simulink model "ejercicio_6d"  (R2020a)
settings: Solver=ode45  StartTime=0.0  StopTime=1  MaxStep=1e-4  RelTol=1e-5
model workspace: external: MATLAB File D:\Ferran\Facultad\UNCuyo\Meca\Automática y Máquinas Eléctricas\Proyecto final\matlab\parametros_y_especs\parametros_y_especif.m (data not in the file)
undefined symbols (not defined in the file): alpha_Cu, beq, Cts, Jeq, L_ls, lambda_m, Ld, Lq, Pp, r, Rref, Rts_amb, sigbuilder_block, Tref
settings Model: Creator=Ferran  LastModifiedBy=Ferran

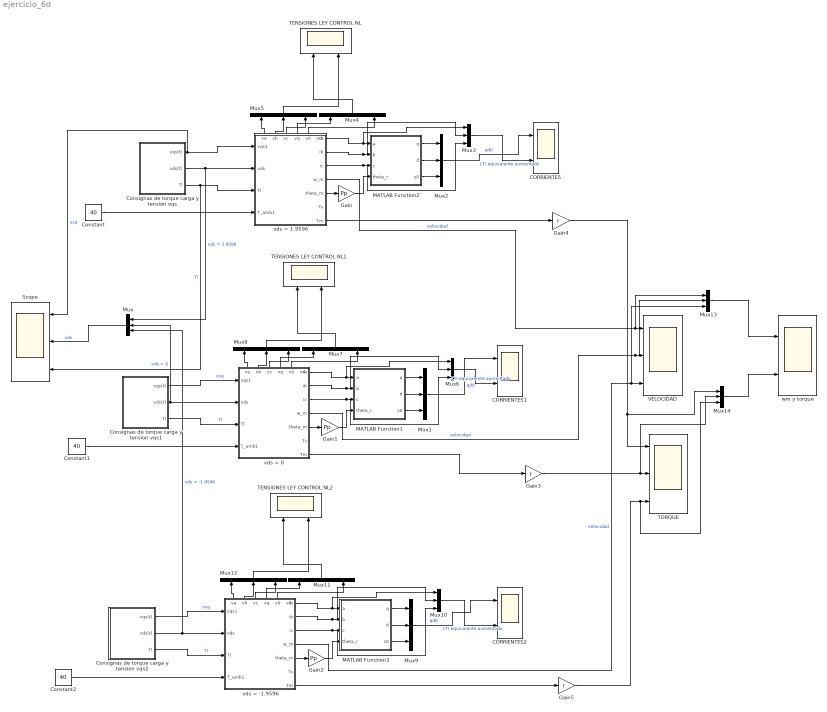
== system ejercicio_6d ==
  CORRIENTES : Scope  NumInputPorts=2
  CORRIENTES1 : Scope  NumInputPorts=2
  CORRIENTES2 : Scope  NumInputPorts=2
  Consignas de torque carga y tension vqs : Subsystem  Tag=STV Subsys  LoadFcn=sigbuilder_block('load');  StartFcn=sigbuilder_block('start');  StopFcn=sigbuilder_block('stop');  ClipboardFcn=sigbuilder_block('clipboard');  mask(Sigbuilder block){tuvar=[0:10]}
      mask help: Simulink:masks:SigbuilderBlock_MD
      mask init:
      | if ~strcmp(get_param(bdroot(gcbh),'SimulationStatus'),'stopped') tuvar = sigbuilder_block('maskInit'); end
      settings: CopyFcn=sigbuilder_block('copy');  DeleteFcn=sigbuilder_block('delete');  ModelCloseFcn=sigbuilder_block('modelClose');  PreSaveFcn=sigbuilder_block('preSave');  PauseFcn=sigbuilder_block('pause');  ContinueFcn=sigbuilder_block('continue');  NameChangeFcn=sigbuilder_block('namechange');  OpenFcn=sigbuilder_block('open',[352.2 100.2 550.8 400.2 ]);  CloseFcn=sigbuilder_block('close');
      mask Display: plot(0, 0, 100, 100,[2, 2, 32, 32, 2], [68, 8, 8, 68, 68],[32, 2], [38, 38], [32, 19, 2],[53, 60, 44], [32, 17, 17, 2],[16, 16, 31, 31]);txt = getActiveGroup(gcbh);text(2, 100, txt,'verticalAlignment', 'top');
  Consignas de torque carga y tension vqs1 : Subsystem  Tag=STV Subsys  LoadFcn=sigbuilder_block('load');  StartFcn=sigbuilder_block('start');  StopFcn=sigbuilder_block('stop');  ClipboardFcn=sigbuilder_block('clipboard');  mask(Sigbuilder block){tuvar=[0:10]}
      mask help: Simulink:masks:SigbuilderBlock_MD
      mask init:
      | if ~strcmp(get_param(bdroot(gcbh),'SimulationStatus'),'stopped') tuvar = sigbuilder_block('maskInit'); end
      settings: CopyFcn=sigbuilder_block('copy');  DeleteFcn=sigbuilder_block('delete');  ModelCloseFcn=sigbuilder_block('modelClose');  PreSaveFcn=sigbuilder_block('preSave');  PauseFcn=sigbuilder_block('pause');  ContinueFcn=sigbuilder_block('continue');  NameChangeFcn=sigbuilder_block('namechange');  OpenFcn=sigbuilder_block('open',[352.2 100.2 550.8 400.2 ]);  CloseFcn=sigbuilder_block('close');
      mask Display: plot(0, 0, 100, 100,[2, 2, 32, 32, 2], [68, 8, 8, 68, 68],[32, 2], [38, 38], [32, 19, 2],[53, 60, 44], [32, 17, 17, 2],[16, 16, 31, 31]);txt = getActiveGroup(gcbh);text(2, 100, txt,'verticalAlignment', 'top');
  Consignas de torque carga y tension vqs2 : Subsystem  Tag=STV Subsys  LoadFcn=sigbuilder_block('load');  StartFcn=sigbuilder_block('start');  StopFcn=sigbuilder_block('stop');  ClipboardFcn=sigbuilder_block('clipboard');  mask(Sigbuilder block){tuvar=[0:10]}
      mask help: Simulink:masks:SigbuilderBlock_MD
      mask init:
      | if ~strcmp(get_param(bdroot(gcbh),'SimulationStatus'),'stopped') tuvar = sigbuilder_block('maskInit'); end
      settings: CopyFcn=sigbuilder_block('copy');  DeleteFcn=sigbuilder_block('delete');  ModelCloseFcn=sigbuilder_block('modelClose');  PreSaveFcn=sigbuilder_block('preSave');  PauseFcn=sigbuilder_block('pause');  ContinueFcn=sigbuilder_block('continue');  NameChangeFcn=sigbuilder_block('namechange');  OpenFcn=sigbuilder_block('open',[352.2 100.2 550.8 400.2 ]);  CloseFcn=sigbuilder_block('close');
      mask Display: plot(0, 0, 100, 100,[2, 2, 32, 32, 2], [68, 8, 8, 68, 68],[32, 2], [38, 38], [32, 19, 2],[53, 60, 44], [32, 17, 17, 2],[16, 16, 31, 31]);txt = getActiveGroup(gcbh);text(2, 100, txt,'verticalAlignment', 'top');
  Constant : Constant  Value=40
  Constant1 : Constant  Value=40
  Constant2 : Constant  Value=40
  Gain : Gain  Gain=Pp
  Gain1 : Gain  Gain=Pp
  Gain2 : Gain  Gain=Pp
  Gain3 : Gain  Gain=r
  Gain4 : Gain  Gain=r
  Gain5 : Gain  Gain=r
  MATLAB Function1 : MATLAB Function  TreatAsAtomicUnit=on
  MATLAB Function2 : MATLAB Function  TreatAsAtomicUnit=on
  MATLAB Function3 : MATLAB Function  TreatAsAtomicUnit=on
  Mux{,1..14} (15 alike) : Mux  Inputs=3
  Scope : Scope  NumInputPorts=3
  TENSIONES LEY CONTROL NL : Scope  NumInputPorts=2
  TENSIONES LEY CONTROL NL1 : Scope  NumInputPorts=2
  TENSIONES LEY CONTROL NL2 : Scope  NumInputPorts=2
  TORQUE : Scope  NumInputPorts=3
  VELOCIDAD : Scope  NumInputPorts=3
  vds = -1.9596 : Subsystem
      settings: PortSchema="{\"entries\":[{\"content\":{\"sides\":[{\"content\":{\"connectorIds\":[\"In1\",\"In2\",\"In3\",\"In4\"]},\"type\":\"ConnectorPlacement.EquallySpacedRectSide\",\"uuid\":\"b8095cac-d600-4a62-9325-3b74ef7eef83\"},{\"content\":{\"connectorIds\":[\"Out1\",\"Out2\",\"Out3\",\"Out4\",\"Out5\",\"Out6\",\"Out7\"],\"side\":\"RIGHT\"},\"type\":\"ConnectorPlacement.EquallySpacedRectSide\",\"uuid\":\"fc0a756d-ae96-4315-bbed-bdc2bfc1e608\"},{\"content\":{\"connectorIds\":[\"Out8\",\"Out9\",\"Out10\",\"Out11\",\"Out12\",\"Out13\"],\"side\":\"TOP\"},\"type\":\"ConnectorPlacement.EquallySpacedRectSide\",\"uuid\":\"afbbfdf4-b2ca-493d-b8c6-50a451d76509\"}]},\"type\":\"ConnectorPlacement.EquallySpacedConnector\",\"uuid\":\"0b98ede1-47d2-4348-94af-35dda2463f57\"}],\"packageUris\":[\"http://schema.mathworks.com/mf0/Connector/19700101\"],\"version\":\"1.0\"}"
  vds = 0 : Subsystem
      settings: PortSchema="{\"entries\":[{\"content\":{\"sides\":[{\"content\":{\"connectorIds\":[\"In1\",\"In2\",\"In3\",\"In4\"]},\"type\":\"ConnectorPlacement.EquallySpacedRectSide\",\"uuid\":\"b8095cac-d600-4a62-9325-3b74ef7eef83\"},{\"content\":{\"connectorIds\":[\"Out1\",\"Out2\",\"Out3\",\"Out4\",\"Out5\",\"Out6\",\"Out7\"],\"side\":\"RIGHT\"},\"type\":\"ConnectorPlacement.EquallySpacedRectSide\",\"uuid\":\"fc0a756d-ae96-4315-bbed-bdc2bfc1e608\"},{\"content\":{\"connectorIds\":[\"Out8\",\"Out9\",\"Out10\",\"Out11\",\"Out12\",\"Out13\"],\"side\":\"TOP\"},\"type\":\"ConnectorPlacement.EquallySpacedRectSide\",\"uuid\":\"afbbfdf4-b2ca-493d-b8c6-50a451d76509\"}]},\"type\":\"ConnectorPlacement.EquallySpacedConnector\",\"uuid\":\"0b98ede1-47d2-4348-94af-35dda2463f57\"}],\"packageUris\":[\"http://schema.mathworks.com/mf0/Connector/19700101\"],\"version\":\"1.0\"}"
  vds = 1.9596 : Subsystem
      settings: PortSchema="{\"entries\":[{\"content\":{\"sides\":[{\"content\":{\"connectorIds\":[\"In1\",\"In2\",\"In3\",\"In4\"]},\"type\":\"ConnectorPlacement.EquallySpacedRectSide\",\"uuid\":\"b8095cac-d600-4a62-9325-3b74ef7eef83\"},{\"content\":{\"connectorIds\":[\"Out1\",\"Out2\",\"Out3\",\"Out4\",\"Out5\",\"Out6\",\"Out7\"],\"side\":\"RIGHT\"},\"type\":\"ConnectorPlacement.EquallySpacedRectSide\",\"uuid\":\"fc0a756d-ae96-4315-bbed-bdc2bfc1e608\"},{\"content\":{\"connectorIds\":[\"Out8\",\"Out9\",\"Out10\",\"Out11\",\"Out12\",\"Out13\"],\"side\":\"TOP\"},\"type\":\"ConnectorPlacement.EquallySpacedRectSide\",\"uuid\":\"afbbfdf4-b2ca-493d-b8c6-50a451d76509\"}]},\"type\":\"ConnectorPlacement.EquallySpacedConnector\",\"uuid\":\"0b98ede1-47d2-4348-94af-35dda2463f57\"}],\"packageUris\":[\"http://schema.mathworks.com/mf0/Connector/19700101\"],\"version\":\"1.0\"}"
  wm y torque : Scope  NumInputPorts=2
  wires:
  Constant/1 -> vds = 1.9596/4(T_amb1)
  Consignas de torque carga y tension vqs/1(vqs(t)) -> Scope/1, vds = 1.9596/1(vqs1)  "vsq"
  Consignas de torque carga y tension vqs/3(Tl) -> Scope/3, vds = 1.9596/3(Tl)  "Tl"
  MATLAB Function2/1(q) -> Mux2/1
  MATLAB Function2/2(d) -> Mux2/2
  MATLAB Function2/3(z0) -> Mux2/3
  vds = 1.9596/11(vq) -> Mux4/1
  vds = 1.9596/12(v0) -> Mux4/3
  Mux4/1 -> TENSIONES LEY CONTROL NL/1
  vds = 1.9596/8(va) -> Mux5/1
  vds = 1.9596/9(vb) -> Mux5/2
  vds = 1.9596/10(vc) -> Mux5/3
  Mux5/1 -> TENSIONES LEY CONTROL NL/2
  Consignas de torque carga y tension vqs/2(vds(t)) -> Mux/1, vds = 1.9596/2(vds)  "vds = 1.9596"
  vds = 1.9596/5(theta_m) -> Gain/1
  Gain/1 -> MATLAB Function2/4(theta_r)
  vds = 1.9596/1(ia) -> Mux3/1, MATLAB Function2/1(a)
  vds = 1.9596/2(ib) -> Mux3/2, MATLAB Function2/2(b)
  vds = 1.9596/3(ic) -> Mux3/3, MATLAB Function2/3(c)
  vds = 0/1(ia) -> Mux6/1, MATLAB Function1/1(a)
  MATLAB Function1/1(q) -> Mux1/1
  vds = 0/3(ic) -> Mux6/3, MATLAB Function1/3(c)
  vds = 0/5(theta_m) -> Gain1/1
  vds = 0/12(v0) -> Mux7/3
  Gain1/1 -> MATLAB Function1/4(theta_r)
  Consignas de torque carga y tension vqs1/2(vds(t)) -> Mux/2, vds = 0/2(vds)  "vds = 0"
  vds = 0/10(vc) -> Mux8/3
  Mux8/1 -> TENSIONES LEY CONTROL NL1/2
  vds = 0/2(ib) -> Mux6/2, MATLAB Function1/2(b)
  vds = 0/9(vb) -> Mux8/2
  Mux7/1 -> TENSIONES LEY CONTROL NL1/1
  vds = 0/11(vq) -> Mux7/1
  vds = 0/8(va) -> Mux8/1
  MATLAB Function1/3(z0) -> Mux1/3
  MATLAB Function1/2(d) -> Mux1/2
  Constant1/1 -> vds = 0/4(T_amb1)
  Consignas de torque carga y tension vqs1/3(Tl) -> vds = 0/3(Tl)  "Tl"
  Consignas de torque carga y tension vqs1/1(vqs(t)) -> vds = 0/1(vqs1)  "vsq"
  vds = -1.9596/1(ia) -> Mux10/1, MATLAB Function3/1(a)
  MATLAB Function3/1(q) -> Mux9/1
  vds = -1.9596/3(ic) -> Mux10/3, MATLAB Function3/3(c)
  vds = -1.9596/5(theta_m) -> Gain2/1
  vds = -1.9596/12(v0) -> Mux11/3
  Gain2/1 -> MATLAB Function3/4(theta_r)
  Consignas de torque carga y tension vqs2/2(vds(t)) -> Mux/3, vds = -1.9596/2(vds)  "vds = -1.9596"
  vds = -1.9596/10(vc) -> Mux12/3
  Mux12/1 -> TENSIONES LEY CONTROL NL2/2
  vds = -1.9596/2(ib) -> Mux10/2, MATLAB Function3/2(b)
  vds = -1.9596/9(vb) -> Mux12/2
  Mux11/1 -> TENSIONES LEY CONTROL NL2/1
  vds = -1.9596/11(vq) -> Mux11/1
  vds = -1.9596/8(va) -> Mux12/1
  MATLAB Function3/3(z0) -> Mux9/3
  MATLAB Function3/2(d) -> Mux9/2
  Constant2/1 -> vds = -1.9596/4(T_amb1)
  Consignas de torque carga y tension vqs2/3(Tl) -> vds = -1.9596/3(Tl)  "Tl"
  Consignas de torque carga y tension vqs2/1(vqs(t)) -> vds = -1.9596/1(vqs1)  "vsq"
  Mux/1 -> Scope/2  "vds"
  vds = 0/4(w_m) -> Mux13/2, VELOCIDAD/2  "velocidad"
  vds = 1.9596/4(w_m) -> Mux13/1, VELOCIDAD/1  "velocidad"
  vds = -1.9596/4(w_m) -> VELOCIDAD/3, Mux13/3  "velocidad"
  vds = 1.9596/7(Tm) -> Gain4/1
  vds = 0/7(Tm) -> Gain3/1
  vds = -1.9596/7(Tm) -> Gain5/1
  Mux13/1 -> wm y torque/1
  Mux14/1 -> wm y torque/2
  Mux3/1 -> CORRIENTES/2  "LTI equivalente aumentado"
  Mux2/1 -> CORRIENTES/1  "qd0"
  Mux6/1 -> CORRIENTES1/2  "LTI equivalente aumentado"
  Mux1/1 -> CORRIENTES1/1  "qd0"
  Mux10/1 -> CORRIENTES2/2  "LTI equivalente aumentado"
  Mux9/1 -> CORRIENTES2/1  "qd0"
  Gain3/1 -> Mux14/2, TORQUE/2
  Gain4/1 -> Mux14/1, TORQUE/1
  Gain5/1 -> Mux14/3, TORQUE/3

== system ejercicio_6d/Consignas de torque carga y tension vqs ==
  Demux : Demux  Tag=STV Demux  Outputs=3
      settings: DisplayOption=none
  FromWs : FromWorkspace  Tag=STV FromWs  VariableName=tuvar
      SigBuilderData=|
      | common.afterFinalStr = 'Extrapolate'
      | common.sampleTime = 0
      | dataSet.timeRange = [0 2]
      | dataSet.name = 'Group 1'
      | sbobj.Groups.Name = 'Group 1'
      | sbobj.Groups.Signals(1).Name = 'vqs(t)'
      | sbobj.Groups.Signals(1).XData = [0 0.1 0.1 0.7 0.7 2]
      | sbobj.Groups.Signals(1).YData = [0 0 19.596 19.596 0 0]
      | sbobj.Groups.Signals(2).Name = 'vds(t)'
      | sbobj.Groups.Signals(2).XData = [0 0.5 0.5 2]
      | sbobj.Groups.Signals(2).YData = [0 0 1.9596 1.9596]
      | sbobj.Groups.Signals(3).Name = 'Tl'
      | sbobj.Groups.Signals(3).XData = [0 0.3 0.3 0.5 0.5 0.9 0.9 2]
      | sbobj.Groups.Signals(3).YData = [0 0 6.28 6.28 -6.28 -6.28 0 0]
      | sbobj.Groups.TimeRange = [0 2]
  vqs(t) : Outport  Tag=STV Outport
  vds(t) : Outport  Tag=STV Outport  Port=2
  Tl : Outport  Tag=STV Outport  Port=3
  wires:
  FromWs/1 -> Demux/1
  Demux/1 -> vqs(t)/1
  Demux/2 -> vds(t)/1
  Demux/3 -> Tl/1

== system ejercicio_6d/Consignas de torque carga y tension vqs1 ==
  Demux : Demux  Tag=STV Demux  Outputs=3
      settings: DisplayOption=none
  FromWs : FromWorkspace  Tag=STV FromWs  VariableName=tuvar
      SigBuilderData=|
      | common.afterFinalStr = 'Extrapolate'
      | common.sampleTime = 0
      | dataSet.timeRange = [0 2]
      | dataSet.name = 'Group 1'
      | sbobj.Groups.Name = 'Group 1'
      | sbobj.Groups.Signals(1).Name = 'vqs(t)'
      | sbobj.Groups.Signals(1).XData = [0 0.1 0.1 0.7 0.7 2]
      | sbobj.Groups.Signals(1).YData = [0 0 19.596 19.596 0 0]
      | sbobj.Groups.Signals(2).Name = 'vds(t)'
      | sbobj.Groups.Signals(2).XData = [0 2]
      | sbobj.Groups.Signals(2).YData = [0 0]
      | sbobj.Groups.Signals(3).Name = 'Tl'
      | sbobj.Groups.Signals(3).XData = [0 0.3 0.3 0.5 0.5 0.9 0.9 2]
      | sbobj.Groups.Signals(3).YData = [0 0 6.28 6.28 -6.28 -6.28 0 0]
      | sbobj.Groups.TimeRange = [0 2]
  vqs(t) : Outport  Tag=STV Outport
  vds(t) : Outport  Tag=STV Outport  Port=2
  Tl : Outport  Tag=STV Outport  Port=3
  wires:
  FromWs/1 -> Demux/1
  Demux/1 -> vqs(t)/1
  Demux/2 -> vds(t)/1
  Demux/3 -> Tl/1

== system ejercicio_6d/Consignas de torque carga y tension vqs2 ==
  Demux : Demux  Tag=STV Demux  Outputs=3
      settings: DisplayOption=none
  FromWs : FromWorkspace  Tag=STV FromWs  VariableName=tuvar
      SigBuilderData=|
      | common.afterFinalStr = 'Extrapolate'
      | common.sampleTime = 0
      | dataSet.timeRange = [0 2]
      | dataSet.name = 'Group 1'
      | sbobj.Groups.Name = 'Group 1'
      | sbobj.Groups.Signals(1).Name = 'vqs(t)'
      | sbobj.Groups.Signals(1).XData = [0 0.1 0.1 0.7 0.7 2]
      | sbobj.Groups.Signals(1).YData = [0 0 19.596 19.596 0 0]
      | sbobj.Groups.Signals(2).Name = 'vds(t)'
      | sbobj.Groups.Signals(2).XData = [0 0.5 0.5 2]
      | sbobj.Groups.Signals(2).YData = [0 0 -1.9596 -1.9596]
      | sbobj.Groups.Signals(3).Name = 'Tl'
      | sbobj.Groups.Signals(3).XData = [0 0.3 0.3 0.5 0.5 0.9 0.9 2]
      | sbobj.Groups.Signals(3).YData = [0 0 6.28 6.28 -6.28 -6.28 0 0]
      | sbobj.Groups.TimeRange = [0 2]
  vqs(t) : Outport  Tag=STV Outport
  vds(t) : Outport  Tag=STV Outport  Port=2
  Tl : Outport  Tag=STV Outport  Port=3
  wires:
  FromWs/1 -> Demux/1
  Demux/1 -> vqs(t)/1
  Demux/2 -> vds(t)/1
  Demux/3 -> Tl/1

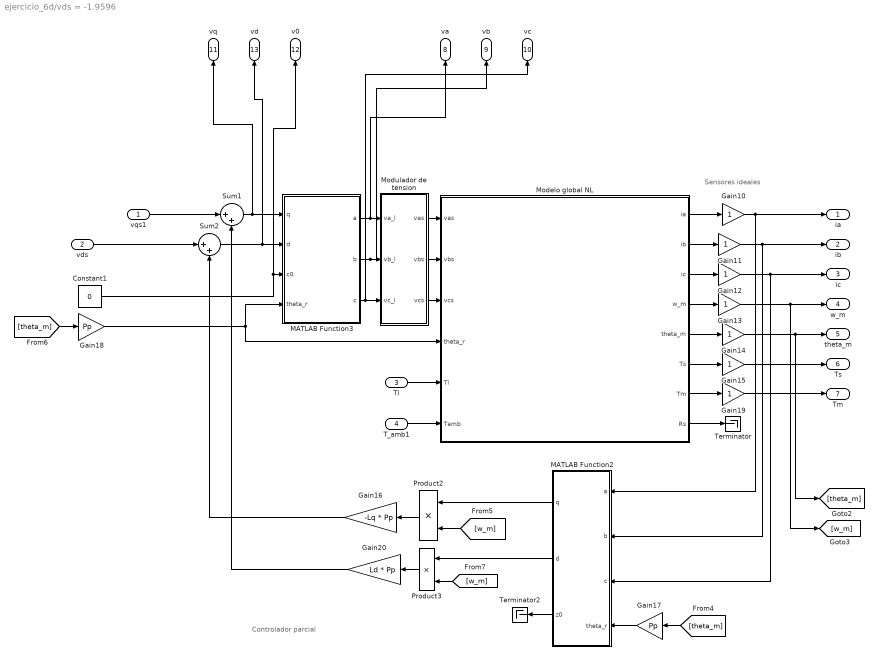
== system ejercicio_6d/vds = -1.9596 ==
  note: Sensores ideales
  note: Controlador parcial
  vqs1 : Inport
  vds : Inport  Port=2
  Tl : Inport  Port=3
  T_amb1 : Inport  Port=4
  Constant1 : Constant  Value=0
  Gain{10..15,19} (7 alike) : Gain
  Gain16 : Gain  Gain=-Lq * Pp
  Gain17 : Gain  Gain=Pp
  Gain18 : Gain  Gain=Pp
  Gain20 : Gain  Gain=Ld * Pp
  MATLAB Function2 : MATLAB Function  TreatAsAtomicUnit=on
  MATLAB Function3 : MATLAB Function  TreatAsAtomicUnit=on
  Modelo global NL : Subsystem
  Modulador de tension : Subsystem
  Product2 : Product
  Product3 : Product
  Sum1 : Sum  Inputs=|++
  Sum2 : Sum  Inputs=|++
  Terminator : Terminator
  Terminator2 : Terminator
  ia : Outport
  ib : Outport  Port=2
  ic : Outport  Port=3
  w_m : Outport  Port=4
  theta_m : Outport  Port=5
  Ts : Outport  Port=6
  Tm : Outport  Port=7
  va : Outport  Port=8
  vb : Outport  Port=9
  vc : Outport  Port=10
  vq : Outport  Port=11
  v0 : Outport  Port=12
  vd : Outport  Port=13
  wires:
  Modelo global NL/2(ib) -> Gain11/1
  MATLAB Function2/3(z0) -> Terminator2/1
  Modelo global NL/8(Rs) -> Terminator/1
  MATLAB Function2/2(d) -> Product3/1
  Modulador de tension/3(vcs) -> Modelo global NL/3(vcs)
  vqs1/1 -> Sum1/1
  Sum1/1 -> vq/1, MATLAB Function3/1(q)
  Constant1/1 -> v0/1, MATLAB Function3/3(c0)
  Gain18/1 -> MATLAB Function3/4(theta_r), Modelo global NL/4(theta_r)
  MATLAB Function3/3(c) -> Modulador de tension/3(vc_l), vc/1
  Gain13/1 -> w_m/1, [w_m]
  Modelo global NL/3(ic) -> Gain12/1
  Modelo global NL/5(theta_m) -> Gain14/1
  Product3/1 -> Gain20/1
  [w_m] -> Product3/2
  Product2/1 -> Gain16/1
  MATLAB Function2/1(q) -> Product2/1
  Modelo global NL/6(Ts) -> Gain15/1
  Gain11/1 -> ib/1, MATLAB Function2/2(b)
  Gain14/1 -> theta_m/1, [theta_m]
  Gain15/1 -> Ts/1
  Gain17/1 -> MATLAB Function2/4(theta_r)
  T_amb1/1 -> Modelo global NL/6(Tamb)
  Modelo global NL/7(Tm) -> Gain19/1
  [theta_m] -> Gain17/1
  [theta_m] -> Gain18/1
  Gain10/1 -> ia/1, MATLAB Function2/1(a)
  MATLAB Function3/1(a) -> va/1, Modulador de tension/1(va_l)
  [w_m] -> Product2/2
  Modulador de tension/1(vas) -> Modelo global NL/1(vas)
  Gain20/1 -> Sum1/2
  Tl/1 -> Modelo global NL/5(Tl)
  Gain19/1 -> Tm/1
  Gain12/1 -> ic/1, MATLAB Function2/3(c)
  MATLAB Function3/2(b) -> vb/1, Modulador de tension/2(vb_l)
  Modulador de tension/2(vbs) -> Modelo global NL/2(vbs)
  Modelo global NL/4(w_m) -> Gain13/1
  Modelo global NL/1(ia) -> Gain10/1
  vds/1 -> Sum2/1
  Sum2/1 -> vd/1, MATLAB Function3/2(d)
  Gain16/1 -> Sum2/2

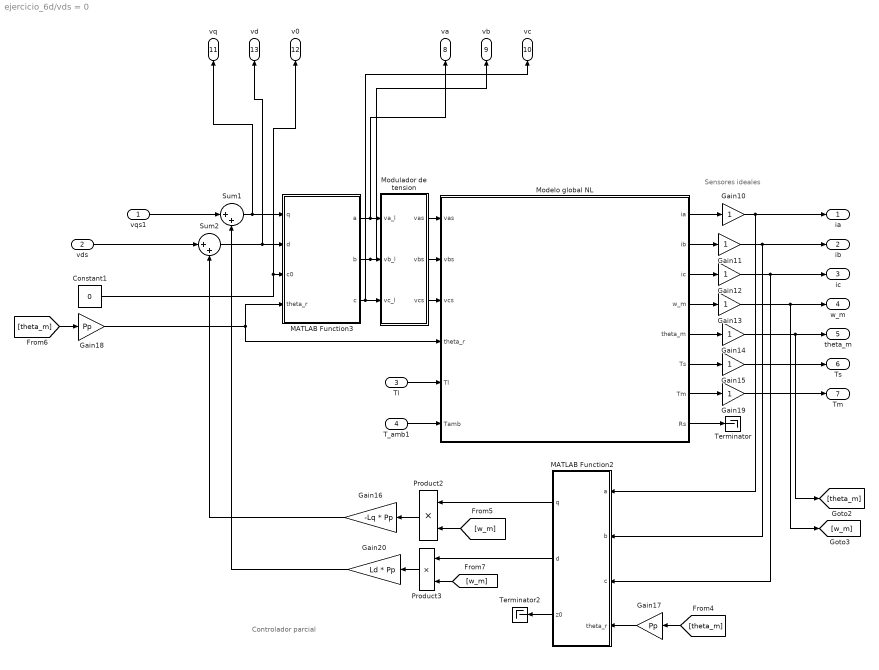
== system ejercicio_6d/vds = 0 ==
  note: Sensores ideales
  note: Controlador parcial
  vqs1 : Inport
  vds : Inport  Port=2
  Tl : Inport  Port=3
  T_amb1 : Inport  Port=4
  Constant1 : Constant  Value=0
  Gain{10..15,19} (7 alike) : Gain
  Gain16 : Gain  Gain=-Lq * Pp
  Gain17 : Gain  Gain=Pp
  Gain18 : Gain  Gain=Pp
  Gain20 : Gain  Gain=Ld * Pp
  MATLAB Function2 : MATLAB Function  TreatAsAtomicUnit=on
  MATLAB Function3 : MATLAB Function  TreatAsAtomicUnit=on
  Modelo global NL : Subsystem
  Modulador de tension : Subsystem
  Product2 : Product
  Product3 : Product
  Sum1 : Sum  Inputs=|++
  Sum2 : Sum  Inputs=|++
  Terminator : Terminator
  Terminator2 : Terminator
  ia : Outport
  ib : Outport  Port=2
  ic : Outport  Port=3
  w_m : Outport  Port=4
  theta_m : Outport  Port=5
  Ts : Outport  Port=6
  Tm : Outport  Port=7
  va : Outport  Port=8
  vb : Outport  Port=9
  vc : Outport  Port=10
  vq : Outport  Port=11
  v0 : Outport  Port=12
  vd : Outport  Port=13
  wires:
  Modelo global NL/2(ib) -> Gain11/1
  MATLAB Function2/3(z0) -> Terminator2/1
  Modelo global NL/8(Rs) -> Terminator/1
  MATLAB Function2/2(d) -> Product3/1
  Modulador de tension/3(vcs) -> Modelo global NL/3(vcs)
  vqs1/1 -> Sum1/1
  Sum1/1 -> vq/1, MATLAB Function3/1(q)
  Constant1/1 -> v0/1, MATLAB Function3/3(c0)
  Gain18/1 -> MATLAB Function3/4(theta_r), Modelo global NL/4(theta_r)
  MATLAB Function3/3(c) -> Modulador de tension/3(vc_l), vc/1
  Gain13/1 -> w_m/1, [w_m]
  Modelo global NL/3(ic) -> Gain12/1
  Modelo global NL/5(theta_m) -> Gain14/1
  Product3/1 -> Gain20/1
  [w_m] -> Product3/2
  Product2/1 -> Gain16/1
  MATLAB Function2/1(q) -> Product2/1
  Modelo global NL/6(Ts) -> Gain15/1
  Gain11/1 -> ib/1, MATLAB Function2/2(b)
  Gain14/1 -> theta_m/1, [theta_m]
  Gain15/1 -> Ts/1
  Gain17/1 -> MATLAB Function2/4(theta_r)
  T_amb1/1 -> Modelo global NL/6(Tamb)
  Modelo global NL/7(Tm) -> Gain19/1
  [theta_m] -> Gain17/1
  [theta_m] -> Gain18/1
  Gain10/1 -> ia/1, MATLAB Function2/1(a)
  MATLAB Function3/1(a) -> va/1, Modulador de tension/1(va_l)
  [w_m] -> Product2/2
  Modulador de tension/1(vas) -> Modelo global NL/1(vas)
  Gain20/1 -> Sum1/2
  Tl/1 -> Modelo global NL/5(Tl)
  Gain19/1 -> Tm/1
  Gain12/1 -> ic/1, MATLAB Function2/3(c)
  MATLAB Function3/2(b) -> vb/1, Modulador de tension/2(vb_l)
  Modulador de tension/2(vbs) -> Modelo global NL/2(vbs)
  Modelo global NL/4(w_m) -> Gain13/1
  Modelo global NL/1(ia) -> Gain10/1
  vds/1 -> Sum2/1
  Sum2/1 -> vd/1, MATLAB Function3/2(d)
  Gain16/1 -> Sum2/2

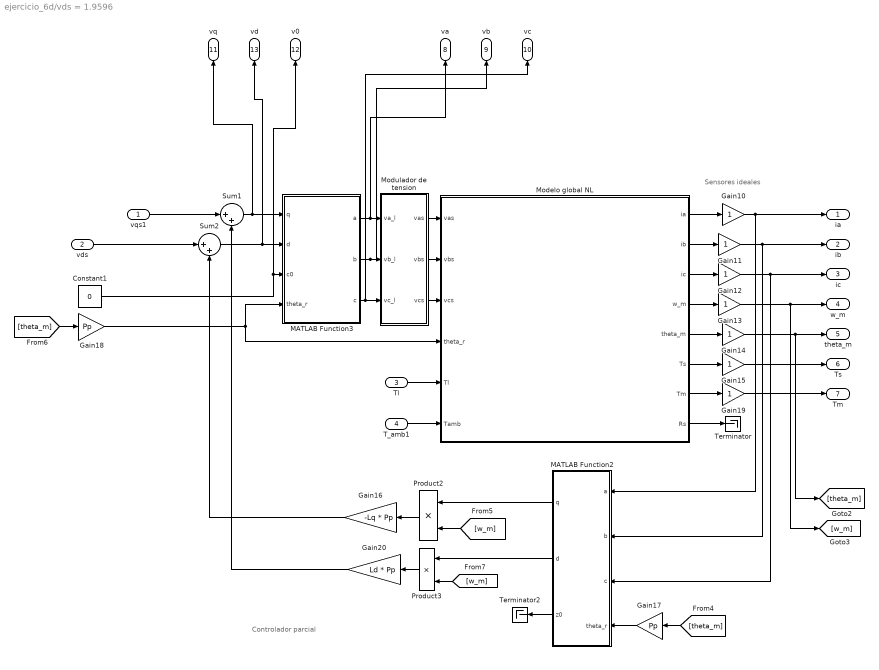
== system ejercicio_6d/vds = 1.9596 ==
  note: Sensores ideales
  note: Controlador parcial
  vqs1 : Inport
  vds : Inport  Port=2
  Tl : Inport  Port=3
  T_amb1 : Inport  Port=4
  Constant1 : Constant  Value=0
  Gain{10..15,19} (7 alike) : Gain
  Gain16 : Gain  Gain=-Lq * Pp
  Gain17 : Gain  Gain=Pp
  Gain18 : Gain  Gain=Pp
  Gain20 : Gain  Gain=Ld * Pp
  MATLAB Function2 : MATLAB Function  TreatAsAtomicUnit=on
  MATLAB Function3 : MATLAB Function  TreatAsAtomicUnit=on
  Modelo global NL : Subsystem
  Modulador de tension : Subsystem
  Product2 : Product
  Product3 : Product
  Sum1 : Sum  Inputs=|++
  Sum2 : Sum  Inputs=|++
  Terminator : Terminator
  Terminator2 : Terminator
  ia : Outport
  ib : Outport  Port=2
  ic : Outport  Port=3
  w_m : Outport  Port=4
  theta_m : Outport  Port=5
  Ts : Outport  Port=6
  Tm : Outport  Port=7
  va : Outport  Port=8
  vb : Outport  Port=9
  vc : Outport  Port=10
  vq : Outport  Port=11
  v0 : Outport  Port=12
  vd : Outport  Port=13
  wires:
  Modelo global NL/2(ib) -> Gain11/1
  MATLAB Function2/3(z0) -> Terminator2/1
  Modelo global NL/8(Rs) -> Terminator/1
  MATLAB Function2/2(d) -> Product3/1
  Modulador de tension/3(vcs) -> Modelo global NL/3(vcs)
  vqs1/1 -> Sum1/1
  Sum1/1 -> vq/1, MATLAB Function3/1(q)
  Constant1/1 -> v0/1, MATLAB Function3/3(c0)
  Gain18/1 -> MATLAB Function3/4(theta_r), Modelo global NL/4(theta_r)
  MATLAB Function3/3(c) -> Modulador de tension/3(vc_l), vc/1
  Gain13/1 -> w_m/1, [w_m]
  Modelo global NL/3(ic) -> Gain12/1
  Modelo global NL/5(theta_m) -> Gain14/1
  Product3/1 -> Gain20/1
  [w_m] -> Product3/2
  Product2/1 -> Gain16/1
  MATLAB Function2/1(q) -> Product2/1
  Modelo global NL/6(Ts) -> Gain15/1
  Gain11/1 -> ib/1, MATLAB Function2/2(b)
  Gain14/1 -> theta_m/1, [theta_m]
  Gain15/1 -> Ts/1
  Gain17/1 -> MATLAB Function2/4(theta_r)
  T_amb1/1 -> Modelo global NL/6(Tamb)
  Modelo global NL/7(Tm) -> Gain19/1
  [theta_m] -> Gain17/1
  [theta_m] -> Gain18/1
  Gain10/1 -> ia/1, MATLAB Function2/1(a)
  MATLAB Function3/1(a) -> va/1, Modulador de tension/1(va_l)
  [w_m] -> Product2/2
  Modulador de tension/1(vas) -> Modelo global NL/1(vas)
  Gain20/1 -> Sum1/2
  Tl/1 -> Modelo global NL/5(Tl)
  Gain19/1 -> Tm/1
  Gain12/1 -> ic/1, MATLAB Function2/3(c)
  MATLAB Function3/2(b) -> vb/1, Modulador de tension/2(vb_l)
  Modulador de tension/2(vbs) -> Modelo global NL/2(vbs)
  Modelo global NL/4(w_m) -> Gain13/1
  Modelo global NL/1(ia) -> Gain10/1
  vds/1 -> Sum2/1
  Sum2/1 -> vd/1, MATLAB Function3/2(d)
  Gain16/1 -> Sum2/2

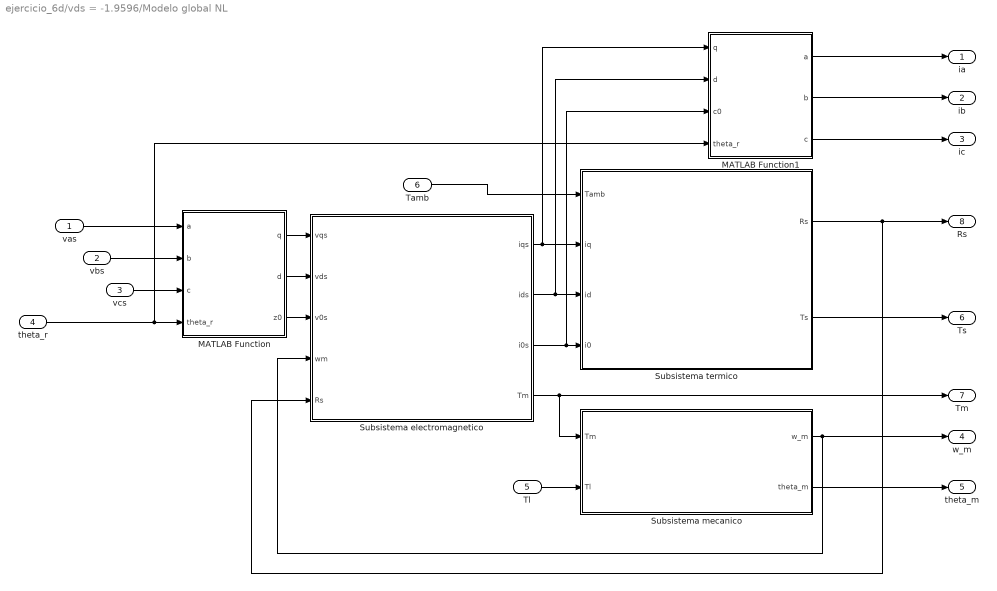
== system ejercicio_6d/vds = -1.9596/Modelo global NL ==
  vas : Inport
  vbs : Inport  Port=2
  vcs : Inport  Port=3
  theta_r : Inport  Port=4
  Tl : Inport  Port=5
  Tamb : Inport  Port=6
  MATLAB Function : MATLAB Function  TreatAsAtomicUnit=on
  MATLAB Function1 : MATLAB Function  TreatAsAtomicUnit=on
  Subsistema electromagnetico : Subsystem
  Subsistema mecanico : Subsystem
  Subsistema termico : Subsystem
  ia : Outport
  ib : Outport  Port=2
  ic : Outport  Port=3
  w_m : Outport  Port=4
  theta_m : Outport  Port=5
  Ts : Outport  Port=6
  Tm : Outport  Port=7
  Rs : Outport  Port=8
  wires:
  MATLAB Function1/3(c) -> ic/1
  MATLAB Function1/2(b) -> ib/1
  Subsistema electromagnetico/4(Tm) -> Tm/1, Subsistema mecanico/1(Tm)
  Subsistema termico/2(Ts) -> Ts/1
  MATLAB Function/1(q) -> Subsistema electromagnetico/1(vqs)
  Subsistema termico/1(Rs) -> Rs/1, Subsistema electromagnetico/5(Rs)
  Subsistema electromagnetico/2(ids) -> MATLAB Function1/2(d), Subsistema termico/3(id)
  Subsistema mecanico/1(w_m) -> w_m/1, Subsistema electromagnetico/4(wm)
  Tamb/1 -> Subsistema termico/1(Tamb)
  Subsistema mecanico/2(theta_m) -> theta_m/1
  MATLAB Function1/1(a) -> ia/1
  Subsistema electromagnetico/1(iqs) -> MATLAB Function1/1(q), Subsistema termico/2(iq)
  vas/1 -> MATLAB Function/1(a)
  Subsistema electromagnetico/3(i0s) -> MATLAB Function1/3(c0), Subsistema termico/4(i0)
  vcs/1 -> MATLAB Function/3(c)
  Tl/1 -> Subsistema mecanico/2(Tl)
  vbs/1 -> MATLAB Function/2(b)
  MATLAB Function/2(d) -> Subsistema electromagnetico/2(vds)
  MATLAB Function/3(z0) -> Subsistema electromagnetico/3(v0s)
  theta_r/1 -> MATLAB Function1/4(theta_r), MATLAB Function/4(theta_r)

== system ejercicio_6d/vds = -1.9596/Modulador de tension ==
  note: Tension de fase
  note: Tension de linea
  va_l : Inport
  vb_l : Inport  Port=2
  vc_l : Inport  Port=3
  Gain1 : Gain
  Gain2 : Gain
  Gain3 : Gain
  vas : Outport
  vbs : Outport  Port=2
  vcs : Outport  Port=3
  wires:
  Gain1/1 -> vbs/1
  va_l/1 -> Gain3/1
  Gain2/1 -> vcs/1
  vb_l/1 -> Gain1/1
  vc_l/1 -> Gain2/1
  Gain3/1 -> vas/1

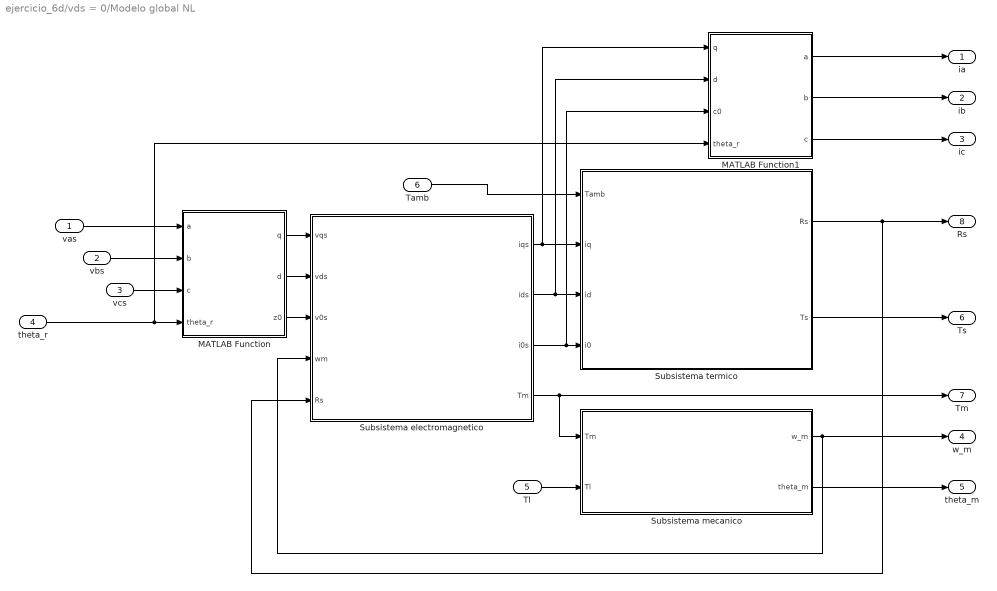
== system ejercicio_6d/vds = 0/Modelo global NL ==
  vas : Inport
  vbs : Inport  Port=2
  vcs : Inport  Port=3
  theta_r : Inport  Port=4
  Tl : Inport  Port=5
  Tamb : Inport  Port=6
  MATLAB Function : MATLAB Function  TreatAsAtomicUnit=on
  MATLAB Function1 : MATLAB Function  TreatAsAtomicUnit=on
  Subsistema electromagnetico : Subsystem
  Subsistema mecanico : Subsystem
  Subsistema termico : Subsystem
  ia : Outport
  ib : Outport  Port=2
  ic : Outport  Port=3
  w_m : Outport  Port=4
  theta_m : Outport  Port=5
  Ts : Outport  Port=6
  Tm : Outport  Port=7
  Rs : Outport  Port=8
  wires:
  MATLAB Function1/3(c) -> ic/1
  MATLAB Function1/2(b) -> ib/1
  Subsistema electromagnetico/4(Tm) -> Tm/1, Subsistema mecanico/1(Tm)
  Subsistema termico/2(Ts) -> Ts/1
  MATLAB Function/1(q) -> Subsistema electromagnetico/1(vqs)
  Subsistema termico/1(Rs) -> Rs/1, Subsistema electromagnetico/5(Rs)
  Subsistema electromagnetico/2(ids) -> MATLAB Function1/2(d), Subsistema termico/3(id)
  Subsistema mecanico/1(w_m) -> w_m/1, Subsistema electromagnetico/4(wm)
  Tamb/1 -> Subsistema termico/1(Tamb)
  Subsistema mecanico/2(theta_m) -> theta_m/1
  MATLAB Function1/1(a) -> ia/1
  Subsistema electromagnetico/1(iqs) -> MATLAB Function1/1(q), Subsistema termico/2(iq)
  vas/1 -> MATLAB Function/1(a)
  Subsistema electromagnetico/3(i0s) -> MATLAB Function1/3(c0), Subsistema termico/4(i0)
  vcs/1 -> MATLAB Function/3(c)
  Tl/1 -> Subsistema mecanico/2(Tl)
  vbs/1 -> MATLAB Function/2(b)
  MATLAB Function/2(d) -> Subsistema electromagnetico/2(vds)
  MATLAB Function/3(z0) -> Subsistema electromagnetico/3(v0s)
  theta_r/1 -> MATLAB Function1/4(theta_r), MATLAB Function/4(theta_r)

== system ejercicio_6d/vds = 0/Modulador de tension ==
  note: Tension de fase
  note: Tension de linea
  va_l : Inport
  vb_l : Inport  Port=2
  vc_l : Inport  Port=3
  Gain1 : Gain
  Gain2 : Gain
  Gain3 : Gain
  vas : Outport
  vbs : Outport  Port=2
  vcs : Outport  Port=3
  wires:
  Gain1/1 -> vbs/1
  va_l/1 -> Gain3/1
  Gain2/1 -> vcs/1
  vb_l/1 -> Gain1/1
  vc_l/1 -> Gain2/1
  Gain3/1 -> vas/1

== system ejercicio_6d/vds = 1.9596/Modelo global NL ==
  vas : Inport
  vbs : Inport  Port=2
  vcs : Inport  Port=3
  theta_r : Inport  Port=4
  Tl : Inport  Port=5
  Tamb : Inport  Port=6
  MATLAB Function : MATLAB Function  TreatAsAtomicUnit=on
  MATLAB Function1 : MATLAB Function  TreatAsAtomicUnit=on
  Subsistema electromagnetico : Subsystem
  Subsistema mecanico : Subsystem
  Subsistema termico : Subsystem
  ia : Outport
  ib : Outport  Port=2
  ic : Outport  Port=3
  w_m : Outport  Port=4
  theta_m : Outport  Port=5
  Ts : Outport  Port=6
  Tm : Outport  Port=7
  Rs : Outport  Port=8
  wires:
  MATLAB Function1/3(c) -> ic/1
  MATLAB Function1/2(b) -> ib/1
  Subsistema electromagnetico/4(Tm) -> Tm/1, Subsistema mecanico/1(Tm)
  Subsistema termico/2(Ts) -> Ts/1
  MATLAB Function/1(q) -> Subsistema electromagnetico/1(vqs)
  Subsistema termico/1(Rs) -> Rs/1, Subsistema electromagnetico/5(Rs)
  Subsistema electromagnetico/2(ids) -> MATLAB Function1/2(d), Subsistema termico/3(id)
  Subsistema mecanico/1(w_m) -> w_m/1, Subsistema electromagnetico/4(wm)
  Tamb/1 -> Subsistema termico/1(Tamb)
  Subsistema mecanico/2(theta_m) -> theta_m/1
  MATLAB Function1/1(a) -> ia/1
  Subsistema electromagnetico/1(iqs) -> MATLAB Function1/1(q), Subsistema termico/2(iq)
  vas/1 -> MATLAB Function/1(a)
  Subsistema electromagnetico/3(i0s) -> MATLAB Function1/3(c0), Subsistema termico/4(i0)
  vcs/1 -> MATLAB Function/3(c)
  Tl/1 -> Subsistema mecanico/2(Tl)
  vbs/1 -> MATLAB Function/2(b)
  MATLAB Function/2(d) -> Subsistema electromagnetico/2(vds)
  MATLAB Function/3(z0) -> Subsistema electromagnetico/3(v0s)
  theta_r/1 -> MATLAB Function1/4(theta_r), MATLAB Function/4(theta_r)

== system ejercicio_6d/vds = 1.9596/Modulador de tension ==
  note: Tension de fase
  note: Tension de linea
  va_l : Inport
  vb_l : Inport  Port=2
  vc_l : Inport  Port=3
  Gain1 : Gain
  Gain2 : Gain
  Gain3 : Gain
  vas : Outport
  vbs : Outport  Port=2
  vcs : Outport  Port=3
  wires:
  Gain1/1 -> vbs/1
  va_l/1 -> Gain3/1
  Gain2/1 -> vcs/1
  vb_l/1 -> Gain1/1
  vc_l/1 -> Gain2/1
  Gain3/1 -> vas/1

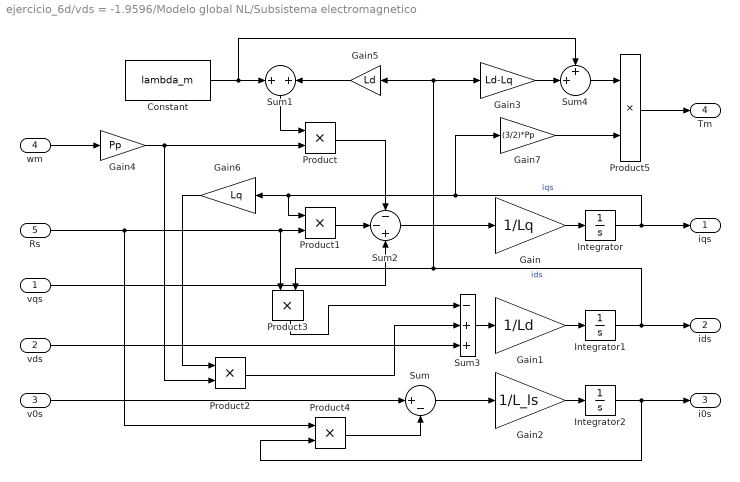
== system ejercicio_6d/vds = -1.9596/Modelo global NL/Subsistema electromagnetico ==
  vqs : Inport
  vds : Inport  Port=2
  v0s : Inport  Port=3
  wm : Inport  Port=4
  Rs : Inport  Port=5
  Constant : Constant  Value=lambda_m
  Gain : Gain  Gain=1/Lq
  Gain1 : Gain  Gain=1/Ld
  Gain2 : Gain  Gain=1/L_ls
  Gain3 : Gain  Gain=Ld-Lq
  Gain4 : Gain  Gain=Pp
  Gain5 : Gain  Gain=Ld
  Gain6 : Gain  Gain=Lq
  Gain7 : Gain  Gain=(3/2)*Pp
  Integrator : Integrator
  Integrator1 : Integrator
  Integrator2 : Integrator
  Product{,1..5} (6 alike) : Product
  Sum : Sum  Inputs=|+-
  Sum1 : Sum  Inputs=+|+
  Sum2 : Sum  Inputs=--+
  Sum3 : Sum  Inputs=-++
  Sum4 : Sum  Inputs=++|
  iqs : Outport
  ids : Outport  Port=2
  i0s : Outport  Port=3
  Tm : Outport  Port=4
  wires:
  Constant/1 -> Sum1/1, Sum4/1
  Product1/1 -> Sum2/2
  Rs/1 -> Product1/2, Product3/1, Product4/1
  Integrator/1 -> iqs/1, Gain7/1, Gain6/1, Product1/1  "iqs"
  Gain3/1 -> Sum4/2
  Sum/1 -> Gain2/1
  Sum2/1 -> Gain/1
  vqs/1 -> Sum2/3
  Product3/1 -> Sum3/1
  Product4/1 -> Sum/2
  vds/1 -> Sum3/3
  Sum3/1 -> Gain1/1
  Gain6/1 -> Product2/1
  Integrator1/1 -> ids/1, Product3/2, Gain5/1, Gain3/1  "ids"
  Product2/1 -> Sum3/2
  Integrator2/1 -> i0s/1, Product4/2
  wm/1 -> Gain4/1
  Sum1/1 -> Product/1
  Gain5/1 -> Sum1/2
  Product/1 -> Sum2/1
  Gain/1 -> Integrator/1
  v0s/1 -> Sum/1
  Gain2/1 -> Integrator2/1
  Gain1/1 -> Integrator1/1
  Gain7/1 -> Product5/2
  Product5/1 -> Tm/1
  Gain4/1 -> Product/2, Product2/2
  Sum4/1 -> Product5/1

== system ejercicio_6d/vds = -1.9596/Modelo global NL/Subsistema mecanico ==
  Tm : Inport
  Tl : Inport  Port=2
  Gain1 : Gain  Gain=1/Jeq
  Gain2 : Gain  Gain=beq
  Gain3 : Gain  Gain=1/r
  Integrator : Integrator
  Integrator1 : Integrator
  Sum : Sum  Inputs=-|+|-
  w_m : Outport
  theta_m : Outport  Port=2
  wires:
  Tm/1 -> Sum/2
  Gain3/1 -> Sum/1
  Integrator/1 -> w_m/1, Gain2/1, Integrator1/1
  Integrator1/1 -> theta_m/1
  Gain2/1 -> Sum/3
  Sum/1 -> Gain1/1
  Tl/1 -> Gain3/1
  Gain1/1 -> Integrator/1

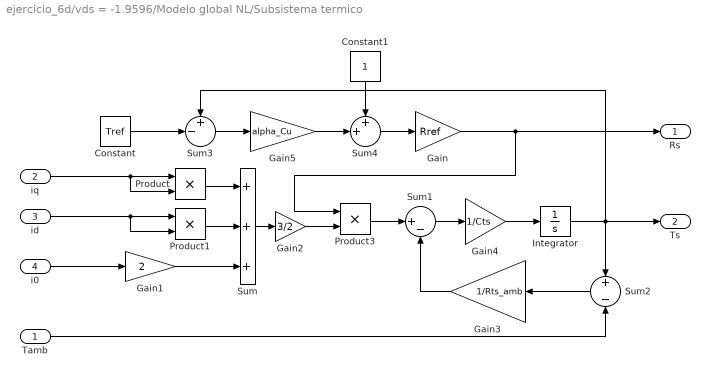
== system ejercicio_6d/vds = -1.9596/Modelo global NL/Subsistema termico ==
  Tamb : Inport
  iq : Inport  Port=2
  id : Inport  Port=3
  i0 : Inport  Port=4
  Constant : Constant  Value=Tref
  Constant1 : Constant
  Gain : Gain  Gain=Rref
  Gain1 : Gain  Gain=2
  Gain2 : Gain  Gain=3/2
  Gain3 : Gain  Gain=1/Rts_amb
  Gain4 : Gain  Gain=1/Cts
  Gain5 : Gain  Gain=alpha_Cu
  Integrator : Integrator  InitialCondition=40
  Product : Product
  Product1 : Product
  Product3 : Product
  Sum : Sum  Inputs=+++
  Sum1 : Sum  Inputs=|+-
  Sum2 : Sum  Inputs=+-
  Sum3 : Sum  Inputs=+-|
  Sum4 : Sum  Inputs=++|
  Rs : Outport
  Ts : Outport  Port=2
  wires:
  Gain1/1 -> Sum/3
  Constant/1 -> Sum3/2
  iq/1 -> Product/1, Product/2
  Product3/1 -> Sum1/1
  Integrator/1 -> Ts/1, Sum3/1, Sum2/1
  Gain4/1 -> Integrator/1
  id/1 -> Product1/1, Product1/2
  Sum3/1 -> Gain5/1
  Constant1/1 -> Sum4/1
  Sum4/1 -> Gain/1
  Gain3/1 -> Sum1/2
  Tamb/1 -> Sum2/2
  Sum1/1 -> Gain4/1
  Gain/1 -> Rs/1, Product3/1
  Product1/1 -> Sum/2
  i0/1 -> Gain1/1
  Gain2/1 -> Product3/2
  Product/1 -> Sum/1
  Gain5/1 -> Sum4/2
  Sum/1 -> Gain2/1
  Sum2/1 -> Gain3/1

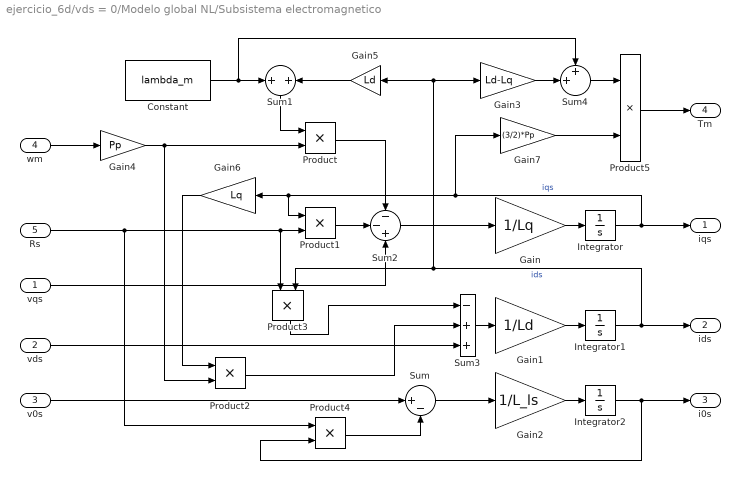
== system ejercicio_6d/vds = 0/Modelo global NL/Subsistema electromagnetico ==
  vqs : Inport
  vds : Inport  Port=2
  v0s : Inport  Port=3
  wm : Inport  Port=4
  Rs : Inport  Port=5
  Constant : Constant  Value=lambda_m
  Gain : Gain  Gain=1/Lq
  Gain1 : Gain  Gain=1/Ld
  Gain2 : Gain  Gain=1/L_ls
  Gain3 : Gain  Gain=Ld-Lq
  Gain4 : Gain  Gain=Pp
  Gain5 : Gain  Gain=Ld
  Gain6 : Gain  Gain=Lq
  Gain7 : Gain  Gain=(3/2)*Pp
  Integrator : Integrator
  Integrator1 : Integrator
  Integrator2 : Integrator
  Product{,1..5} (6 alike) : Product
  Sum : Sum  Inputs=|+-
  Sum1 : Sum  Inputs=+|+
  Sum2 : Sum  Inputs=--+
  Sum3 : Sum  Inputs=-++
  Sum4 : Sum  Inputs=++|
  iqs : Outport
  ids : Outport  Port=2
  i0s : Outport  Port=3
  Tm : Outport  Port=4
  wires:
  Constant/1 -> Sum1/1, Sum4/1
  Product1/1 -> Sum2/2
  Rs/1 -> Product1/2, Product3/1, Product4/1
  Integrator/1 -> iqs/1, Gain7/1, Gain6/1, Product1/1  "iqs"
  Gain3/1 -> Sum4/2
  Sum/1 -> Gain2/1
  Sum2/1 -> Gain/1
  vqs/1 -> Sum2/3
  Product3/1 -> Sum3/1
  Product4/1 -> Sum/2
  vds/1 -> Sum3/3
  Sum3/1 -> Gain1/1
  Gain6/1 -> Product2/1
  Integrator1/1 -> ids/1, Product3/2, Gain5/1, Gain3/1  "ids"
  Product2/1 -> Sum3/2
  Integrator2/1 -> i0s/1, Product4/2
  wm/1 -> Gain4/1
  Sum1/1 -> Product/1
  Gain5/1 -> Sum1/2
  Product/1 -> Sum2/1
  Gain/1 -> Integrator/1
  v0s/1 -> Sum/1
  Gain2/1 -> Integrator2/1
  Gain1/1 -> Integrator1/1
  Gain7/1 -> Product5/2
  Product5/1 -> Tm/1
  Gain4/1 -> Product/2, Product2/2
  Sum4/1 -> Product5/1

== system ejercicio_6d/vds = 0/Modelo global NL/Subsistema mecanico ==
  Tm : Inport
  Tl : Inport  Port=2
  Gain1 : Gain  Gain=1/Jeq
  Gain2 : Gain  Gain=beq
  Gain3 : Gain  Gain=1/r
  Integrator : Integrator
  Integrator1 : Integrator
  Sum : Sum  Inputs=-|+|-
  w_m : Outport
  theta_m : Outport  Port=2
  wires:
  Tm/1 -> Sum/2
  Gain3/1 -> Sum/1
  Integrator/1 -> w_m/1, Gain2/1, Integrator1/1
  Integrator1/1 -> theta_m/1
  Gain2/1 -> Sum/3
  Sum/1 -> Gain1/1
  Tl/1 -> Gain3/1
  Gain1/1 -> Integrator/1

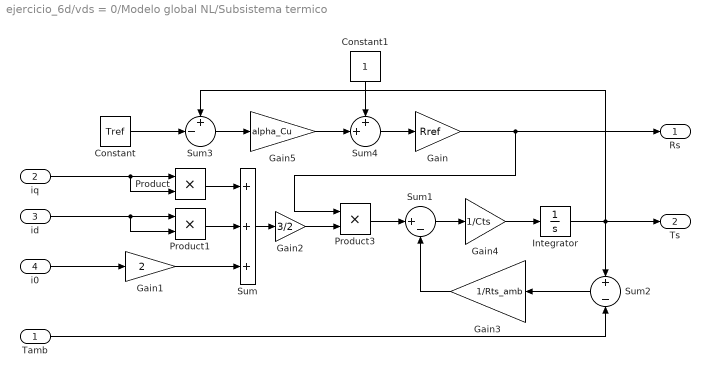
== system ejercicio_6d/vds = 0/Modelo global NL/Subsistema termico ==
  Tamb : Inport
  iq : Inport  Port=2
  id : Inport  Port=3
  i0 : Inport  Port=4
  Constant : Constant  Value=Tref
  Constant1 : Constant
  Gain : Gain  Gain=Rref
  Gain1 : Gain  Gain=2
  Gain2 : Gain  Gain=3/2
  Gain3 : Gain  Gain=1/Rts_amb
  Gain4 : Gain  Gain=1/Cts
  Gain5 : Gain  Gain=alpha_Cu
  Integrator : Integrator  InitialCondition=40
  Product : Product
  Product1 : Product
  Product3 : Product
  Sum : Sum  Inputs=+++
  Sum1 : Sum  Inputs=|+-
  Sum2 : Sum  Inputs=+-
  Sum3 : Sum  Inputs=+-|
  Sum4 : Sum  Inputs=++|
  Rs : Outport
  Ts : Outport  Port=2
  wires:
  Gain1/1 -> Sum/3
  Constant/1 -> Sum3/2
  iq/1 -> Product/1, Product/2
  Product3/1 -> Sum1/1
  Integrator/1 -> Ts/1, Sum3/1, Sum2/1
  Gain4/1 -> Integrator/1
  id/1 -> Product1/1, Product1/2
  Sum3/1 -> Gain5/1
  Constant1/1 -> Sum4/1
  Sum4/1 -> Gain/1
  Gain3/1 -> Sum1/2
  Tamb/1 -> Sum2/2
  Sum1/1 -> Gain4/1
  Gain/1 -> Rs/1, Product3/1
  Product1/1 -> Sum/2
  i0/1 -> Gain1/1
  Gain2/1 -> Product3/2
  Product/1 -> Sum/1
  Gain5/1 -> Sum4/2
  Sum/1 -> Gain2/1
  Sum2/1 -> Gain3/1

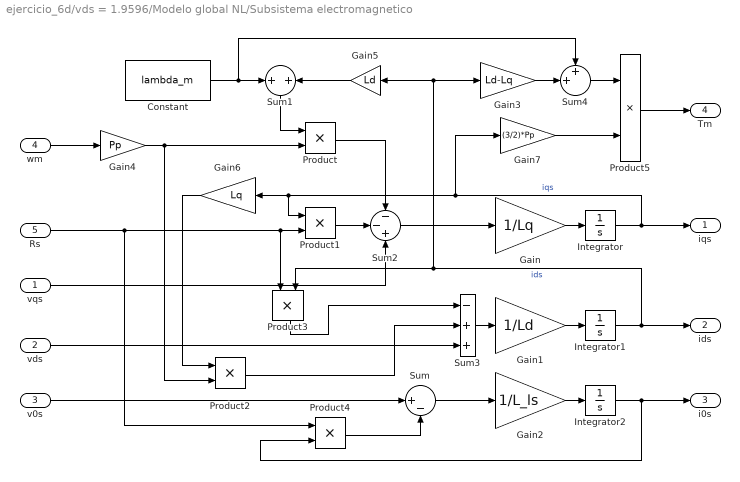
== system ejercicio_6d/vds = 1.9596/Modelo global NL/Subsistema electromagnetico ==
  vqs : Inport
  vds : Inport  Port=2
  v0s : Inport  Port=3
  wm : Inport  Port=4
  Rs : Inport  Port=5
  Constant : Constant  Value=lambda_m
  Gain : Gain  Gain=1/Lq
  Gain1 : Gain  Gain=1/Ld
  Gain2 : Gain  Gain=1/L_ls
  Gain3 : Gain  Gain=Ld-Lq
  Gain4 : Gain  Gain=Pp
  Gain5 : Gain  Gain=Ld
  Gain6 : Gain  Gain=Lq
  Gain7 : Gain  Gain=(3/2)*Pp
  Integrator : Integrator
  Integrator1 : Integrator
  Integrator2 : Integrator
  Product{,1..5} (6 alike) : Product
  Sum : Sum  Inputs=|+-
  Sum1 : Sum  Inputs=+|+
  Sum2 : Sum  Inputs=--+
  Sum3 : Sum  Inputs=-++
  Sum4 : Sum  Inputs=++|
  iqs : Outport
  ids : Outport  Port=2
  i0s : Outport  Port=3
  Tm : Outport  Port=4
  wires:
  Constant/1 -> Sum1/1, Sum4/1
  Product1/1 -> Sum2/2
  Rs/1 -> Product1/2, Product3/1, Product4/1
  Integrator/1 -> iqs/1, Gain7/1, Gain6/1, Product1/1  "iqs"
  Gain3/1 -> Sum4/2
  Sum/1 -> Gain2/1
  Sum2/1 -> Gain/1
  vqs/1 -> Sum2/3
  Product3/1 -> Sum3/1
  Product4/1 -> Sum/2
  vds/1 -> Sum3/3
  Sum3/1 -> Gain1/1
  Gain6/1 -> Product2/1
  Integrator1/1 -> ids/1, Product3/2, Gain5/1, Gain3/1  "ids"
  Product2/1 -> Sum3/2
  Integrator2/1 -> i0s/1, Product4/2
  wm/1 -> Gain4/1
  Sum1/1 -> Product/1
  Gain5/1 -> Sum1/2
  Product/1 -> Sum2/1
  Gain/1 -> Integrator/1
  v0s/1 -> Sum/1
  Gain2/1 -> Integrator2/1
  Gain1/1 -> Integrator1/1
  Gain7/1 -> Product5/2
  Product5/1 -> Tm/1
  Gain4/1 -> Product/2, Product2/2
  Sum4/1 -> Product5/1

== system ejercicio_6d/vds = 1.9596/Modelo global NL/Subsistema mecanico ==
  Tm : Inport
  Tl : Inport  Port=2
  Gain1 : Gain  Gain=1/Jeq
  Gain2 : Gain  Gain=beq
  Gain3 : Gain  Gain=1/r
  Integrator : Integrator
  Integrator1 : Integrator
  Sum : Sum  Inputs=-|+|-
  w_m : Outport
  theta_m : Outport  Port=2
  wires:
  Tm/1 -> Sum/2
  Gain3/1 -> Sum/1
  Integrator/1 -> w_m/1, Gain2/1, Integrator1/1
  Integrator1/1 -> theta_m/1
  Gain2/1 -> Sum/3
  Sum/1 -> Gain1/1
  Tl/1 -> Gain3/1
  Gain1/1 -> Integrator/1

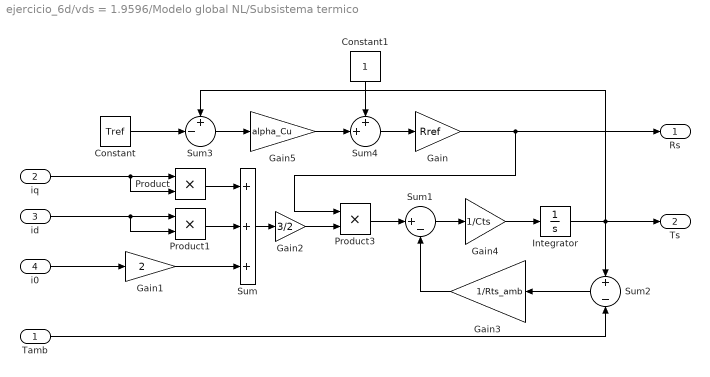
== system ejercicio_6d/vds = 1.9596/Modelo global NL/Subsistema termico ==
  Tamb : Inport
  iq : Inport  Port=2
  id : Inport  Port=3
  i0 : Inport  Port=4
  Constant : Constant  Value=Tref
  Constant1 : Constant
  Gain : Gain  Gain=Rref
  Gain1 : Gain  Gain=2
  Gain2 : Gain  Gain=3/2
  Gain3 : Gain  Gain=1/Rts_amb
  Gain4 : Gain  Gain=1/Cts
  Gain5 : Gain  Gain=alpha_Cu
  Integrator : Integrator  InitialCondition=40
  Product : Product
  Product1 : Product
  Product3 : Product
  Sum : Sum  Inputs=+++
  Sum1 : Sum  Inputs=|+-
  Sum2 : Sum  Inputs=+-
  Sum3 : Sum  Inputs=+-|
  Sum4 : Sum  Inputs=++|
  Rs : Outport
  Ts : Outport  Port=2
  wires:
  Gain1/1 -> Sum/3
  Constant/1 -> Sum3/2
  iq/1 -> Product/1, Product/2
  Product3/1 -> Sum1/1
  Integrator/1 -> Ts/1, Sum3/1, Sum2/1
  Gain4/1 -> Integrator/1
  id/1 -> Product1/1, Product1/2
  Sum3/1 -> Gain5/1
  Constant1/1 -> Sum4/1
  Sum4/1 -> Gain/1
  Gain3/1 -> Sum1/2
  Tamb/1 -> Sum2/2
  Sum1/1 -> Gain4/1
  Gain/1 -> Rs/1, Product3/1
  Product1/1 -> Sum/2
  i0/1 -> Gain1/1
  Gain2/1 -> Product3/2
  Product/1 -> Sum/1
  Gain5/1 -> Sum4/2
  Sum/1 -> Gain2/1
  Sum2/1 -> Gain3/1

== matlab function ejercicio_6d/vds = 0/Modelo global NL/MATLAB Function ==
  data: a input; q output; b input; c input; theta_r input; d output; z0 output
function [q,d,z0] = TPark_directa(a,b,c,theta_r)
    fabc = [a;b;c];
    T = (2/3) * ...
        [ cos(theta_r) cos(theta_r - (2*pi)/3) cos(theta_r + (2*pi)/3);
        sin(theta_r) sin(theta_r - (2*pi)/3) sin(theta_r + (2*pi)/3);
        1/2                   1/2                  1/2];
  
  fqd0 = T*fabc;
  q = fqd0(1);
  d = fqd0(2);
  z0 = fqd0(3);
end

== matlab function ejercicio_6d/vds = 0/Modelo global NL/MATLAB Function1 ==
  data: q input; a output; d input; c0 input; theta_r input; b output; c output
function [a,b,c] = TPark_inversa(q,d,c0,theta_r)
    fqd0 = [q;d;c0];
    T = [cos(theta_r)               sin(theta_r)            1;
        cos(theta_r - (2*pi)/3)    sin(theta_r - (2*pi)/3) 1;
        cos(theta_r + (2*pi)/3)    sin(theta_r + (2*pi)/3) 1];
    
    fabc = T*fqd0;
    
    a = fabc(1);
    b = fabc(2);
    c = fabc(3);
end

== matlab function ejercicio_6d/vds = 1.9596/Modelo global NL/MATLAB Function1 ==
  data: q input; a output; d input; c0 input; theta_r input; b output; c output
function [a,b,c] = TPark_inversa(q,d,c0,theta_r)
    fqd0 = [q;d;c0];
    T = [cos(theta_r)               sin(theta_r)            1;
        cos(theta_r - (2*pi)/3)    sin(theta_r - (2*pi)/3) 1;
        cos(theta_r + (2*pi)/3)    sin(theta_r + (2*pi)/3) 1];
    
    fabc = T*fqd0;
    
    a = fabc(1);
    b = fabc(2);
    c = fabc(3);
end

== matlab function ejercicio_6d/MATLAB Function3 ==
  data: a input; q output; b input; c input; theta_r input; d output; z0 output
function [q,d,z0] = TPark_directa(a,b,c,theta_r)
    fabc = [a;b;c];
    T = (2/3) * ...
        [ cos(theta_r) cos(theta_r - (2*pi)/3) cos(theta_r + (2*pi)/3);
        sin(theta_r) sin(theta_r - (2*pi)/3) sin(theta_r + (2*pi)/3);
        1/2                   1/2                  1/2];
  
  fqd0 = T*fabc;
  q = fqd0(1);
  d = fqd0(2);
  z0 = fqd0(3);
end

== matlab function ejercicio_6d/vds = -1.9596/MATLAB Function2 ==
  data: a input; q output; b input; c input; theta_r input; d output; z0 output
function [q,d,z0] = TPark_directa(a,b,c,theta_r)
    fabc = [a;b;c];
    T = (2/3) * ...
        [ cos(theta_r) cos(theta_r - (2*pi)/3) cos(theta_r + (2*pi)/3);
        sin(theta_r) sin(theta_r - (2*pi)/3) sin(theta_r + (2*pi)/3);
        1/2                   1/2                  1/2];
  
  fqd0 = T*fabc;
  q = fqd0(1);
  d = fqd0(2);
  z0 = fqd0(3);
end

== matlab function ejercicio_6d/vds = -1.9596/MATLAB Function3 ==
  data: q input; a output; d input; c0 input; theta_r input; b output; c output
function [a,b,c] = TPark_inversa(q,d,c0,theta_r)
    fqd0 = [q;d;c0];
    T = [cos(theta_r)               sin(theta_r)            1;
        cos(theta_r - (2*pi)/3)    sin(theta_r - (2*pi)/3) 1;
        cos(theta_r + (2*pi)/3)    sin(theta_r + (2*pi)/3) 1];
    
    fabc = T*fqd0;
    
    a = fabc(1);
    b = fabc(2);
    c = fabc(3);
end

== matlab function ejercicio_6d/vds = -1.9596/Modelo global NL/MATLAB Function ==
  data: a input; q output; b input; c input; theta_r input; d output; z0 output
function [q,d,z0] = TPark_directa(a,b,c,theta_r)
    fabc = [a;b;c];
    T = (2/3) * ...
        [ cos(theta_r) cos(theta_r - (2*pi)/3) cos(theta_r + (2*pi)/3);
        sin(theta_r) sin(theta_r - (2*pi)/3) sin(theta_r + (2*pi)/3);
        1/2                   1/2                  1/2];
  
  fqd0 = T*fabc;
  q = fqd0(1);
  d = fqd0(2);
  z0 = fqd0(3);
end

== matlab function ejercicio_6d/vds = -1.9596/Modelo global NL/MATLAB Function1 ==
  data: q input; a output; d input; c0 input; theta_r input; b output; c output
function [a,b,c] = TPark_inversa(q,d,c0,theta_r)
    fqd0 = [q;d;c0];
    T = [cos(theta_r)               sin(theta_r)            1;
        cos(theta_r - (2*pi)/3)    sin(theta_r - (2*pi)/3) 1;
        cos(theta_r + (2*pi)/3)    sin(theta_r + (2*pi)/3) 1];
    
    fabc = T*fqd0;
    
    a = fabc(1);
    b = fabc(2);
    c = fabc(3);
end

== matlab function ejercicio_6d/vds = 1.9596/Modelo global NL/MATLAB Function ==
  data: a input; q output; b input; c input; theta_r input; d output; z0 output
function [q,d,z0] = TPark_directa(a,b,c,theta_r)
    fabc = [a;b;c];
    T = (2/3) * ...
        [ cos(theta_r) cos(theta_r - (2*pi)/3) cos(theta_r + (2*pi)/3);
        sin(theta_r) sin(theta_r - (2*pi)/3) sin(theta_r + (2*pi)/3);
        1/2                   1/2                  1/2];
  
  fqd0 = T*fabc;
  q = fqd0(1);
  d = fqd0(2);
  z0 = fqd0(3);
end

== matlab function ejercicio_6d/MATLAB Function1 ==
  data: a input; q output; b input; c input; theta_r input; d output; z0 output
function [q,d,z0] = TPark_directa(a,b,c,theta_r)
    fabc = [a;b;c];
    T = (2/3) * ...
        [ cos(theta_r) cos(theta_r - (2*pi)/3) cos(theta_r + (2*pi)/3);
        sin(theta_r) sin(theta_r - (2*pi)/3) sin(theta_r + (2*pi)/3);
        1/2                   1/2                  1/2];
  
  fqd0 = T*fabc;
  q = fqd0(1);
  d = fqd0(2);
  z0 = fqd0(3);
end

== matlab function ejercicio_6d/MATLAB Function2 ==
  data: a input; q output; b input; c input; theta_r input; d output; z0 output
function [q,d,z0] = TPark_directa(a,b,c,theta_r)
    fabc = [a;b;c];
    T = (2/3) * ...
        [ cos(theta_r) cos(theta_r - (2*pi)/3) cos(theta_r + (2*pi)/3);
        sin(theta_r) sin(theta_r - (2*pi)/3) sin(theta_r + (2*pi)/3);
        1/2                   1/2                  1/2];
  
  fqd0 = T*fabc;
  q = fqd0(1);
  d = fqd0(2);
  z0 = fqd0(3);
end

== matlab function ejercicio_6d/vds = 1.9596/MATLAB Function2 ==
  data: a input; q output; b input; c input; theta_r input; d output; z0 output
function [q,d,z0] = TPark_directa(a,b,c,theta_r)
    fabc = [a;b;c];
    T = (2/3) * ...
        [ cos(theta_r) cos(theta_r - (2*pi)/3) cos(theta_r + (2*pi)/3);
        sin(theta_r) sin(theta_r - (2*pi)/3) sin(theta_r + (2*pi)/3);
        1/2                   1/2                  1/2];
  
  fqd0 = T*fabc;
  q = fqd0(1);
  d = fqd0(2);
  z0 = fqd0(3);
end

== matlab function ejercicio_6d/vds = 1.9596/MATLAB Function3 ==
  data: q input; a output; d input; c0 input; theta_r input; b output; c output
function [a,b,c] = TPark_inversa(q,d,c0,theta_r)
    fqd0 = [q;d;c0];
    T = [cos(theta_r)               sin(theta_r)            1;
        cos(theta_r - (2*pi)/3)    sin(theta_r - (2*pi)/3) 1;
        cos(theta_r + (2*pi)/3)    sin(theta_r + (2*pi)/3) 1];
    
    fabc = T*fqd0;
    
    a = fabc(1);
    b = fabc(2);
    c = fabc(3);
end

== matlab function ejercicio_6d/vds = 0/MATLAB Function2 ==
  data: a input; q output; b input; c input; theta_r input; d output; z0 output
function [q,d,z0] = TPark_directa(a,b,c,theta_r)
    fabc = [a;b;c];
    T = (2/3) * ...
        [ cos(theta_r) cos(theta_r - (2*pi)/3) cos(theta_r + (2*pi)/3);
        sin(theta_r) sin(theta_r - (2*pi)/3) sin(theta_r + (2*pi)/3);
        1/2                   1/2                  1/2];
  
  fqd0 = T*fabc;
  q = fqd0(1);
  d = fqd0(2);
  z0 = fqd0(3);
end

== matlab function ejercicio_6d/vds = 0/MATLAB Function3 ==
  data: q input; a output; d input; c0 input; theta_r input; b output; c output
function [a,b,c] = TPark_inversa(q,d,c0,theta_r)
    fqd0 = [q;d;c0];
    T = [cos(theta_r)               sin(theta_r)            1;
        cos(theta_r - (2*pi)/3)    sin(theta_r - (2*pi)/3) 1;
        cos(theta_r + (2*pi)/3)    sin(theta_r + (2*pi)/3) 1];
    
    fabc = T*fqd0;
    
    a = fabc(1);
    b = fabc(2);
    c = fabc(3);
end
